simulink model "receive_nad_r2016b"  (R2016b)
settings: Solver=VariableStepAuto  StartTime=0.0  StopTime=10.0  RelTol=1e-3
libraries: lib_ed247 x2
settings Model: Creator=odufour  LastModifiedBy=odufour
settings DataIOCC: ExternalInput=ds  ReturnWorkspaceOutputs=on
settings DebuggingCC: InheritedTsInSrcMsg=none
settings SFSimCC: SimUseLocalCustomCode=on
settings RTWCC: RTWUseLocalCustomCode=on

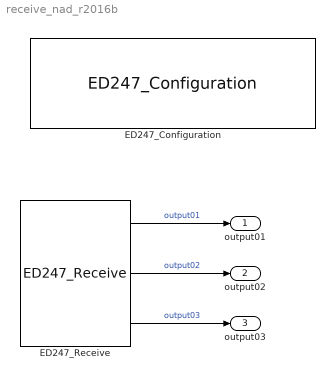
== system receive_nad_r2016b ==
  ED247_Configuration : lib_ed247/ED247_Configuration  configurationFilename='ecic_func_exchange_nad_mc_tester.xml'  enableLog=off  logFilename=''
  ED247_Receive : lib_ed247/ED247_Receive  SFunctionModules=''
  output01 : Outport  OutDataTypeStr=uint8
  output02 : Outport  Port=2  OutDataTypeStr=uint8
  output03 : Outport  Port=3  OutDataTypeStr=single  PortDimensions=[2,2]
  wires:
  ED247_Receive/1 -> output01/1  "output01"
  ED247_Receive/2 -> output02/1  "output02"
  ED247_Receive/3 -> output03/1  "output03"
